simulink model "sys4"  (Simulink 7.3)
settings: Solver=ode45  StartTime=0.0  StopTime=30  MaxStep=0.01  RelTol=1e-3
model workspace (MAT data in the model file):
  ctrl.name = 'ctrl'
  ctrl.type = 'mamdani'
  ctrl.andMethod = 'prod'
  ctrl.orMethod = 'probor'
  ctrl.defuzzMethod = 'centroid'
  ctrl.impMethod = 'prod'
  ctrl.aggMethod = 'sum'
  ctrl.input(1).name = 'E'
  ctrl.input(1).range = [-1 1]
  ctrl.input(1).mf(1).name = 'Negative Large'
  ctrl.input(1).mf(1).type = 'trapmf'
  ctrl.input(1).mf(1).params = [-1 -1 -0.8 0.4]
  ctrl.input(1).mf(2).name = 'Negative'
  ctrl.input(1).mf(2).type = 'trimf'
  ctrl.input(1).mf(2).params = [-0.8 -0.2 -0.01]
  ctrl.input(1).mf(3).name = 'Zero'
  ctrl.input(1).mf(3).type = 'trimf'
  ctrl.input(1).mf(3).params = [0 0 0]
  ctrl.input(1).mf(4).name = 'Positive'
  ctrl.input(1).mf(4).type = 'trimf'
  ctrl.input(1).mf(4).params = [0.01 0.2 0.8]
  ctrl.input(1).mf(5).name = 'Positive Large'
  ctrl.input(1).mf(5).type = 'trapmf'
  ctrl.input(1).mf(5).params = [-0.4 0.8 1 1]
  ctrl.input(2).name = 'CE'
  ctrl.input(2).range = [-1 1]
  ctrl.input(2).mf(1).name = 'Negative Large'
  ctrl.input(2).mf(1).type = 'trapmf'
  ctrl.input(2).mf(1).params = [-1 -1 -0.8 0.4]
  ctrl.input(2).mf(2).name = 'Negative'
  ctrl.input(2).mf(2).type = 'trimf'
  ctrl.input(2).mf(2).params = [-0.8 -0.2 -0.01]
  ctrl.input(2).mf(3).name = 'Zero'
  ctrl.input(2).mf(3).type = 'trimf'
  ctrl.input(2).mf(3).params = [0 0 0]
  ctrl.input(2).mf(4).name = 'Positive'
  ctrl.input(2).mf(4).type = 'trimf'
  ctrl.input(2).mf(4).params = [0.01 0.2 0.8]
  ctrl.input(2).mf(5).name = 'Positive Large'
  ctrl.input(2).mf(5).type = 'trapmf'
  ctrl.input(2).mf(5).params = [-0.4 0.8 1 1]
  ctrl.output.name = 'u'
  ctrl.output.range = [-1 1]
  ctrl.output.mf(1).name = 'LargeNegative'
  ctrl.output.mf(1).type = 'trapmf'
  ctrl.output.mf(1).params = [-1 -1 -0.7 -0.2]
  ctrl.output.mf(2).name = 'SmallNegative'
  ctrl.output.mf(2).type = 'trimf'
  ctrl.output.mf(2).params = [-0.5 -0.2 -0.01]
  ctrl.output.mf(3).name = 'Zero'
  ctrl.output.mf(3).type = 'trimf'
  ctrl.output.mf(3).params = [0 0 0]
  ctrl.output.mf(4).name = 'SmallPositive'
  ctrl.output.mf(4).type = 'trimf'
  ctrl.output.mf(4).params = [0.01 0.2 0.5]
  ctrl.output.mf(5).name = 'LargePositive'
  ctrl.output.mf(5).type = 'trapmf'
  ctrl.output.mf(5).params = [0.2 0.7 1 1]
  ctrl.rule(1).antecedent = [1 1]
  ctrl.rule(1).consequent = 1
  ctrl.rule(1).weight = 1
  ctrl.rule(1).connection = 1
  ctrl.rule(2).antecedent = [1 2]
  ctrl.rule(2).consequent = 1
  ctrl.rule(2).weight = 1
  ctrl.rule(2).connection = 1
  ctrl.rule(3).antecedent = [1 3]
  ctrl.rule(3).consequent = 2
  ctrl.rule(3).weight = 1
  ctrl.rule(3).connection = 1
  ctrl.rule(4).antecedent = [1 4]
  ctrl.rule(4).consequent = 2
  ctrl.rule(4).weight = 1
  ctrl.rule(4).connection = 1
  ctrl.rule(5).antecedent = [1 5]
  ctrl.rule(5).consequent = 3
  ctrl.rule(5).weight = 1
  ctrl.rule(5).connection = 1
  ctrl.rule(6).antecedent = [2 1]
  ctrl.rule(6).consequent = 1
  ctrl.rule(6).weight = 1
  ctrl.rule(6).connection = 1
  ctrl.rule(7).antecedent = [2 2]
  ctrl.rule(7).consequent = 2
  ctrl.rule(7).weight = 1
  ctrl.rule(7).connection = 1
  ctrl.rule(8).antecedent = [2 3]
  ctrl.rule(8).consequent = 2
  ctrl.rule(8).weight = 1
  ctrl.rule(8).connection = 1
  ctrl.rule(9).antecedent = [2 4]
  ctrl.rule(9).consequent = 3
  ctrl.rule(9).weight = 1
  ctrl.rule(9).connection = 1
  ctrl.rule(10).antecedent = [2 5]
  ctrl.rule(10).consequent = 4
  ctrl.rule(10).weight = 1
  ctrl.rule(10).connection = 1
  ctrl.rule(11).antecedent = [3 1]
  ctrl.rule(11).consequent = 2
  ctrl.rule(11).weight = 1
  ctrl.rule(11).connection = 1
  ctrl.rule(12).antecedent = [3 2]
  ctrl.rule(12).consequent = 2
  ctrl.rule(12).weight = 1
  ctrl.rule(12).connection = 1
  ctrl.rule(13).antecedent = [3 3]
  ctrl.rule(13).consequent = 3
  ctrl.rule(13).weight = 1
  ctrl.rule(13).connection = 1
  ctrl.rule(14).antecedent = [3 4]
  ctrl.rule(14).consequent = 4
  ctrl.rule(14).weight = 1
  ctrl.rule(14).connection = 1
  ctrl.rule(15).antecedent = [3 5]
  ctrl.rule(15).consequent = 4
  ctrl.rule(15).weight = 1
  ctrl.rule(15).connection = 1
  ctrl.rule(16).antecedent = [4 1]
  ctrl.rule(16).consequent = 2
  ctrl.rule(16).weight = 1
  ctrl.rule(16).connection = 1
  ctrl.rule(17).antecedent = [4 2]
  ctrl.rule(17).consequent = 3
  ctrl.rule(17).weight = 1
  ctrl.rule(17).connection = 1
  ctrl.rule(18).antecedent = [4 3]
  ctrl.rule(18).consequent = 4
  ctrl.rule(18).weight = 1
  ctrl.rule(18).connection = 1
  ctrl.rule(19).antecedent = [4 4]
  ctrl.rule(19).consequent = 4
  ctrl.rule(19).weight = 1
  ctrl.rule(19).connection = 1
  ctrl.rule(20).antecedent = [4 5]
  ctrl.rule(20).consequent = 5
  ctrl.rule(20).weight = 1
  ctrl.rule(20).connection = 1
  ctrl.rule(21).antecedent = [5 1]
  ctrl.rule(21).consequent = 3
  ctrl.rule(21).weight = 1
  ctrl.rule(21).connection = 1
  ctrl.rule(22).antecedent = [5 2]
  ctrl.rule(22).consequent = 4
  ctrl.rule(22).weight = 1
  ctrl.rule(22).connection = 1
  ctrl.rule(23).antecedent = [5 3]
  ctrl.rule(23).consequent = 4
  ctrl.rule(23).weight = 1
  ctrl.rule(23).connection = 1
  ctrl.rule(24).antecedent = [5 4]
  ctrl.rule(24).consequent = 5
  ctrl.rule(24).weight = 1
  ctrl.rule(24).connection = 1
  ctrl.rule(25).antecedent = [5 5]
  ctrl.rule(25).consequent = 5
  ctrl.rule(25).weight = 1
  ctrl.rule(25).connection : numeric (value not decoded)
libraries: fuzblock x1
settings Model: Creator=srikanth  LastModifiedBy=srikanth

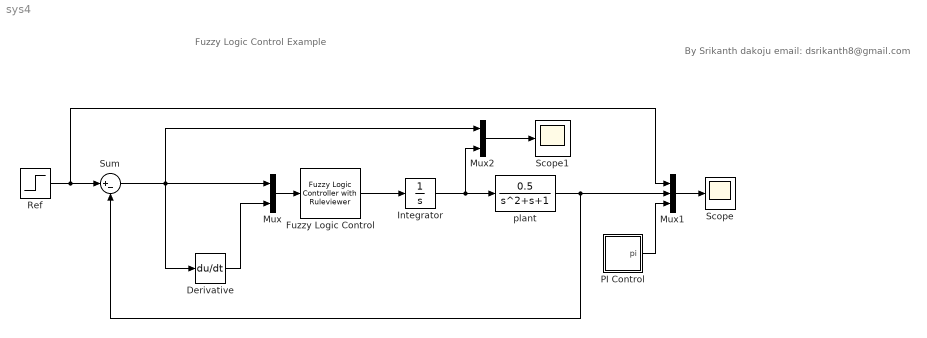
== system sys4 ==
  note: Fuzzy Logic Control Example
  note: By
      | Srikanth dakoju
      | email: dsrikanth8@gmail.com
  Derivative : Derivative  LinearizePole=0.01
  Fuzzy Logic Control : fuzblock/Fuzzy Logic  Controller  with Ruleviewer  SystemSampleTime=-1  fismatrix=ctrl  Ts=2
  Integrator : Integrator
  Mux : Mux  Inputs=2
  Mux1 : Mux  Inputs=3
  Mux2 : Mux  Inputs=2
  PI Control : Subsystem
  Ref : Step  SampleTime=0
  Scope : Scope
      settings: TimeRange=30  YMin=0  YMax=1.4
  Scope1 : Scope
      settings: TimeRange=30  YMin=-0.5  YMax=2.5  SaveName=ScopeData4
  Sum : Sum  Inputs=|+-  OutDataType=fixdt(1, 16)  OutScaling=2^0
  plant : TransferFcn  Numerator=[0.5]  Denominator=[1 1 1]
  wires:
  Mux/1 -> Fuzzy Logic Control/1
  Derivative/1 -> Mux/2
  Sum/1 -> Mux/1, Derivative/1, Mux2/1
  plant/1 -> Sum/2, Mux1/2
  Ref/1 -> Sum/1, Mux1/1
  PI Control/1(pi) -> Mux1/3
  Mux1/1 -> Scope/1
  Mux2/1 -> Scope1/1
  Integrator/1 -> plant/1, Mux2/2
  Fuzzy Logic Control/1 -> Integrator/1

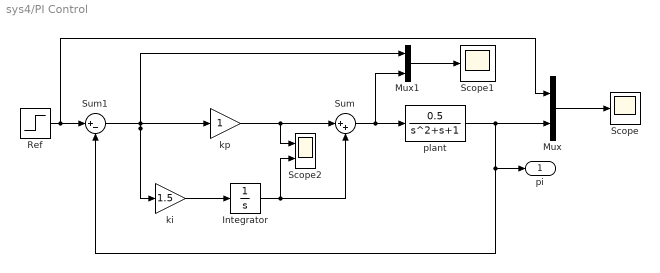
== system sys4/PI Control ==
  Integrator : Integrator
  Mux : Mux  Inputs=2
  Mux1 : Mux  Inputs=2
  Ref : Step  SampleTime=0
  Scope : Scope
      settings: TimeRange=30  YMin=0  YMax=1.4  SaveName=ScopeData3
  Scope1 : Scope
      settings: TimeRange=30  YMin=-0.5  YMax=2.5
  Scope2 : Scope  NumInputPorts=2
      settings: TimeRange=30  YMin=-0.5~-5  YMax=2.5~5  SaveName=ScopeData2
  Sum : Sum  Inputs=|++  OutDataType=fixdt(1, 16)  OutScaling=2^0
  Sum1 : Sum  Inputs=|+-  OutDataType=fixdt(1, 16)  OutScaling=2^0
  ki : Gain  Gain=1.5  ParameterDataType=fixdt(1, 16)  ParameterScaling=2^0  OutDataType=fixdt(1, 16)  OutScaling=2^0
  kp : Gain  ParameterDataType=fixdt(1, 16)  ParameterScaling=2^0  OutDataType=fixdt(1, 16)  OutScaling=2^0
  plant : TransferFcn  Numerator=[0.5]  Denominator=[1 1 1]
  pi : Outport
  wires:
  plant/1 -> Mux/2, Sum1/2, pi/1
  Sum/1 -> plant/1, Mux1/2
  kp/1 -> Sum/1, Scope2/1
  ki/1 -> Integrator/1
  Integrator/1 -> Sum/2, Scope2/2
  Sum1/1 -> kp/1, ki/1, Mux1/1
  Ref/1 -> Sum1/1, Mux/1
  Mux1/1 -> Scope1/1
  Mux/1 -> Scope/1
